simulink model "Jb_Model"  (R2023a)
settings: Solver=VariableStepAuto  StartTime=0.0  StopTime=SimulationTime  RelTol=1e-3
values from neighbouring files (symbols this model uses):
  b = J/taumecc    (= 0.000861176470588)    [BaseModelForControl_Parameters_DAHLIN.m]    (also in BaseModelForControl_Parameters_DEADBEAT.m; BaseModelForControl_Parameters_ESTIM.m; BaseModelForControl_Parameters_PI.m; DAHLINModel_Parameters.m = 0.00085764)
  bstim = cast(bstim,"double")    [Jb_estimation_DCMotor.m]
  J = Jdc+Jbr    (= 7.32e-05)    [BaseModelForControl_Parameters_DAHLIN.m]    (also in BaseModelForControl_Parameters_DEADBEAT.m; BaseModelForControl_Parameters_ESTIM.m; BaseModelForControl_Parameters_PI.m; DAHLINModel_Parameters.m = 8.3561e-05)
  Jstim = cast(Jstim,"double")    [Jb_estimation_DCMotor.m]
  TSample = PWM_Period    (= 0.0001)    [BaseModelForControl_Parameters_DAHLIN.m]    (also in BaseModelForControl_Parameters_DEADBEAT.m; BaseModelForControl_Parameters_ESTIM.m; BaseModelForControl_Parameters_PI.m; DAHLINModel_Parameters.m)
settings Model: Creator=Davide  LastModifiedBy=Teo Santini
settings DataIOCC: ReturnWorkspaceOutputs=off
settings OptimizationCC: ReuseModelBlockBuffer=off

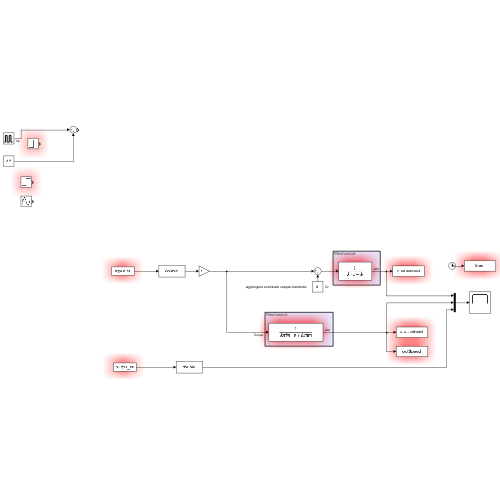
[thumbnail: Simulink's stored preview of the top-level diagram]
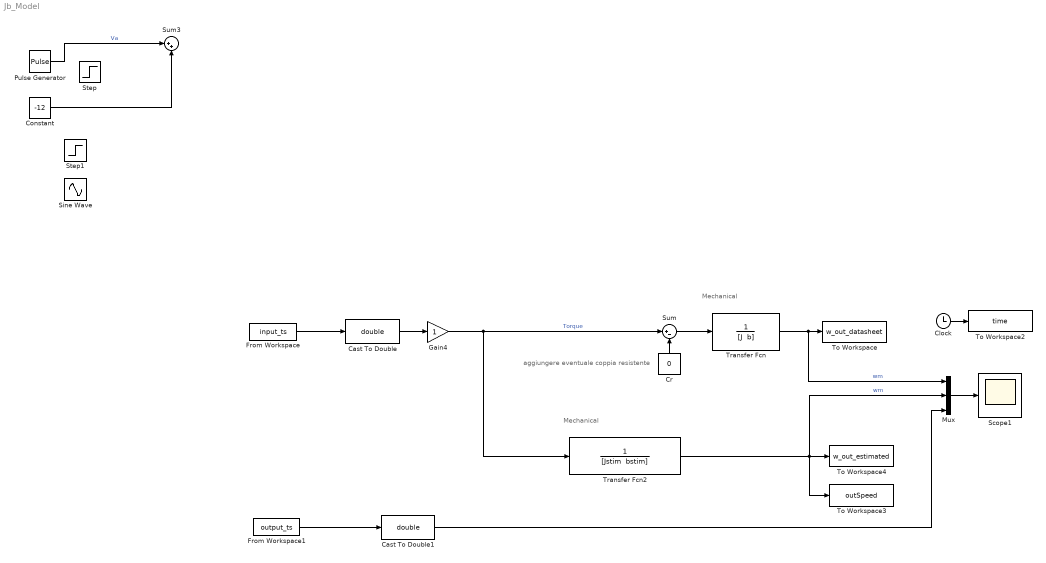
== system Jb_Model ==
  note: aggiungere eventuale coppia resistente
  note: Mechanical
  note: Mechanical
  Cast To Double : DataTypeConversion  OutDataTypeStr=double  SaturateOnIntegerOverflow=off  RndMeth=Floor
  Cast To Double1 : DataTypeConversion  OutDataTypeStr=double  SaturateOnIntegerOverflow=off  RndMeth=Floor
  Clock : Clock
  Constant : Constant  Value=-12
  Cr : Constant  Value=0
  From Workspace : FromWorkspace  VariableName=input_ts  SampleTime=TSample
  From Workspace1 : FromWorkspace  VariableName=output_ts  SampleTime=TSample
  Gain4 : Gain
  Mux : Mux  Inputs=3
  Pulse Generator : DiscretePulseGenerator  PulseType=Time based  Amplitude=24  Period=1  PulseWidth=20  PhaseDelay=-0.002
  Scope1 : Scope
  Sine Wave : Sin  Amplitude=12  Frequency=150  SampleTime=0
  Step : Step  Time=0  After=24  SampleTime=TSample
  Step1 : Step  Time=0  After=24  SampleTime=TSample
  Sum : Sum  Inputs=|+-
  Sum3 : Sum  Inputs=|++
  To Workspace : ToWorkspace  VariableName=w_out_datasheet  SampleTime=TSample
  To Workspace2 : ToWorkspace  VariableName=time  SampleTime=TSample
  To Workspace3 : ToWorkspace  VariableName=outSpeed  SampleTime=TSample
  To Workspace4 : ToWorkspace  VariableName=w_out_estimated  SampleTime=TSample
  Transfer Fcn : TransferFcn  Denominator="[J  b]"
  Transfer Fcn2 : TransferFcn  Denominator="[Jstim  bstim]"
  wires:
  Transfer Fcn/1 -> Mux/1, To Workspace/1  "wm"
  Gain4/1 -> Transfer Fcn2/1, Sum/1  "Torque"
  Transfer Fcn2/1 -> To Workspace3/1, To Workspace4/1, Mux/2  "wm"
  Mux/1 -> Scope1/1
  Sum/1 -> Transfer Fcn/1
  Clock/1 -> To Workspace2/1
  Constant/1 -> Sum3/2
  From Workspace/1 -> Cast To Double/1
  Pulse Generator/1 -> Sum3/1  "Va"
  Cast To Double/1 -> Gain4/1
  From Workspace1/1 -> Cast To Double1/1
  Cast To Double1/1 -> Mux/3
  Cr/1 -> Sum/2
